simulink library "wt_blockset_v3"  (Simulink 6.0)
settings: Solver=ode45  SolverMode=SingleTasking  StartTime=0.0  StopTime=10.0  RelTol=1e-3
undefined symbols (not defined in the file): f1, get, j, Kmode, Type, u0
libraries: simulink_extras x12, simulink3 x5, simulink x4, dspinverses x1, dspmtrx3 x1, dspsnks4 x1
(part 4 of 7)

== system wt_blockset_v3/Control/WT Controller 2 MW DFIG/Pitch System ==
  In : Inport  Port=1  LatchInput=off
  Rate Limiter : RateLimiter  RisingSlewLimit=8  FallingSlewLimit=-8
  Saturation1 : Saturate  UpperLimit=90  LowerLimit=-90
  Out : Outport
  wires:
  Rate Limiter/1 -> Saturation1/1
  In/1 -> Rate Limiter/1
  Saturation1/1 -> Out/1

== system wt_blockset_v3/Control/WT Controller 2 MW DFIG/Power Controller ==
  Ref : Inport  Port=1  LatchInput=off
  Meas : Inport  Port=2  LatchInput=off
  Gain : Inport  Port=3  LatchInput=off
  1/T : Gain  Gain=1/Ti  SaturateOnIntegerOverflow=on
  Integrator : Integrator  InitialCondition=init_cond
  Limit Pitch : Saturate  UpperLimit=24  LowerLimit=0
  P1 : Gain  Gain=K  SaturateOnIntegerOverflow=on
  P2 : Gain  Orientation=left  Gain=ka  SaturateOnIntegerOverflow=on
  Product : Product  InputSameDT=on
  Sum1 : Sum  Inputs=|+-  SaturateOnIntegerOverflow=on  InputSameDT=on
  Sum2 : Sum  Inputs=++|  SaturateOnIntegerOverflow=on  InputSameDT=on
  Sum3 : Sum  Inputs=|+-  SaturateOnIntegerOverflow=on  InputSameDT=on
  Sum4 : Sum  Orientation=left  Inputs=+-|  SaturateOnIntegerOverflow=on  InputSameDT=on
  Out : Outport  InitialOutput=0
  wires:
  Limit Pitch/1 -> Sum4/2, Out/1
  Sum4/1 -> P2/1
  Sum2/1 -> Limit Pitch/1, Sum4/1
  P2/1 -> Sum1/2
  Meas/1 -> Sum3/2
  Ref/1 -> Sum3/1
  Sum3/1 -> P1/1
  1/T/1 -> Integrator/1
  Integrator/1 -> Sum2/2
  Sum1/1 -> 1/T/1
  P1/1 -> Product/1
  Product/1 -> Sum1/1, Sum2/1
  Gain/1 -> Product/2

== system wt_blockset_v3/Control/WT Controller 2 MW DFIG/Speed Controller ==
  ref : Inport  Port=1  LatchInput=off
  meas : Inport  Port=2  LatchInput=off
  1/T : Gain  Gain=1/Ti  SaturateOnIntegerOverflow=on
  Integrator : Integrator  InitialCondition=init_cond
  P1 : Gain  Gain=K  SaturateOnIntegerOverflow=on
  P2 : Gain  Orientation=left  Gain=ka  SaturateOnIntegerOverflow=on
  Saturation : Saturate  UpperLimit=maxim  LowerLimit=-maxim
  Sum1 : Sum  Inputs=|+-  SaturateOnIntegerOverflow=on  InputSameDT=on
  Sum2 : Sum  Inputs=++|  SaturateOnIntegerOverflow=on  InputSameDT=on
  Sum3 : Sum  Inputs=|+-  SaturateOnIntegerOverflow=on  InputSameDT=on
  Sum4 : Sum  Orientation=left  Inputs=+-|  SaturateOnIntegerOverflow=on  InputSameDT=on
  out : Outport  InitialOutput=0
  wires:
  Saturation/1 -> Sum4/2, out/1
  Sum4/1 -> P2/1
  Sum2/1 -> Saturation/1, Sum4/1
  P2/1 -> Sum1/2
  meas/1 -> Sum3/2
  P1/1 -> Sum2/1, Sum1/1
  ref/1 -> Sum3/1
  Sum3/1 -> P1/1
  1/T/1 -> Integrator/1
  Integrator/1 -> Sum2/2
  Sum1/1 -> 1/T/1

== system wt_blockset_v3/Electrical Machinery/C S-Function based  Models/ABC/abc Squirrel Cage Induction Machine ==
  us_UVW : Inport  Port=1  LatchInput=off
  omg_mec : Inport  Port=2  LatchInput=off
  Connection Type : Constant  Value=Type
  Demux : Demux  Outputs=[3 1]
  Mux : Mux  Inputs=[3 1]
  S-Function : S-Function  FunctionName=abc_scim_zcs  Parameters=stator rotor Lm p x0_init
  Switch : Switch  SaturateOnIntegerOverflow=on  InputSameDT=on
  mode : Gain  Gain=Kmode  SaturateOnIntegerOverflow=on
  phase ->line : Subsystem
  is_UVW : Outport
  Te : Outport  Port=2
  wires:
  Mux/1 -> S-Function/1
  S-Function/1 -> Demux/1
  us_UVW/1 -> mode/1
  omg_mec/1 -> Mux/2
  Demux/2 -> Te/1
  mode/1 -> Mux/1
  phase ->line/1(Out) -> Switch/3
  Connection Type/1 -> Switch/2
  Switch/1 -> is_UVW/1
  Demux/1 -> Switch/1, phase ->line/1(In)

== system wt_blockset_v3/Electrical Machinery/C S-Function based  Models/ABC/abc Wound Rotor Induction Machine ==
  us_UVW : Inport  Port=1  LatchInput=off
  ur_KLM : Inport  Port=2  LatchInput=off
  omg_mec : Inport  Port=3  LatchInput=off
  Connection Type : Constant  Value=Type
  Demux : Demux  Outputs=[3 3 1]
  Mux : Mux  Inputs=[3 3 1]
  S-Function : S-Function  FunctionName=abc_wrim_zcs  Parameters=stator rotor Lm p x0_init
  Switch : Switch  SaturateOnIntegerOverflow=on  InputSameDT=on
  mode : Gain  Gain=Kmode  SaturateOnIntegerOverflow=on
  phase ->line1 : Subsystem
  is_UVW : Outport
  ir_KLM : Outport  Port=2
  Te : Outport  Port=3
  wires:
  Mux/1 -> S-Function/1
  S-Function/1 -> Demux/1
  us_UVW/1 -> mode/1
  mode/1 -> Mux/1
  phase ->line1/1(Out) -> Switch/3
  Connection Type/1 -> Switch/2
  Switch/1 -> is_UVW/1
  Demux/1 -> Switch/1, phase ->line1/1(In)
  omg_mec/1 -> Mux/3
  ur_KLM/1 -> Mux/2
  Demux/3 -> Te/1
  Demux/2 -> ir_KLM/1

== system wt_blockset_v3/Electrical Machinery/C S-Function based  Models/DQ Salient-Pole Synchronous Machine ==
  us_UVW : Inport  Port=1  LatchInput=off
  uf : Inport  Port=2  LatchInput=off
  omg_mec : Inport  Port=3  LatchInput=off
  Demux : Demux  Outputs=[3 1 1]
  Mux : Mux  Inputs=[3 1 1]
  S-Function : S-Function  FunctionName=sp_sm_rot_mask  Parameters=stator_winding, field_winding, rotor_winding, mag_ind, p
  is_UVW : Outport  InitialOutput=0
  if : Outport  Port=2  InitialOutput=0
  Te : Outport  Port=3  InitialOutput=0
  wires:
  us_UVW/1 -> Mux/1
  uf/1 -> Mux/2
  omg_mec/1 -> Mux/3
  Demux/1 -> is_UVW/1
  Demux/2 -> if/1
  Demux/3 -> Te/1
  Mux/1 -> S-Function/1
  S-Function/1 -> Demux/1

== system wt_blockset_v3/Electrical Machinery/C S-Function based  Models/DQ Squirrel Cage Induction Machine ==
  us_UVW : Inport  Port=1  LatchInput=off
  omg_mec : Inport  Port=2  LatchInput=off
  Demux : Demux  Outputs=[3 1]
  Mux : Mux  Inputs=[3 1]
  S-Function : S-Function  FunctionName=dq_scim  Parameters=stator rotor Lm p x0_init
  is_UVW : Outport
  Te : Outport  Port=2
  wires:
  Demux/2 -> Te/1
  Demux/1 -> is_UVW/1
  omg_mec/1 -> Mux/2
  us_UVW/1 -> Mux/1
  S-Function/1 -> Demux/1
  Mux/1 -> S-Function/1

== system wt_blockset_v3/Electrical Machinery/C S-Function based  Models/DQ Wound Rotor Induction Machine ==
  us_UVW : Inport  Port=1  LatchInput=off
  ur_KLM : Inport  Port=2  LatchInput=off
  omg_mec : Inport  Port=3  LatchInput=off
  Demux : Demux  Outputs=[3 3 1]
  Mux : Mux  Inputs=[3 3 1]
  S-Function : S-Function  FunctionName=wr_imr  Parameters=stator rotor Lm p x0_init
  is_UVW : Outport
  ir_KLM : Outport  Port=2
  Te : Outport  Port=3
  wires:
  Demux/3 -> Te/1
  Demux/2 -> ir_KLM/1
  Demux/1 -> is_UVW/1
  omg_mec/1 -> Mux/3
  ur_KLM/1 -> Mux/2
  us_UVW/1 -> Mux/1
  S-Function/1 -> Demux/1
  Mux/1 -> S-Function/1

== system wt_blockset_v3/Electrical Machinery/Simulink Blocks  based Models/ABC/abc Squirell-Cage Induction Machine ==
  v_UVW : Inport  Port=1  LatchInput=off
  omg_mec : Inport  Port=2  LatchInput=off
  Connection Type : Constant  Value=Type
  Int_iA : Integrator  InitialCondition=init_cond(1)
  Int_iB : Integrator  InitialCondition=init_cond(2)
  Int_iC : Integrator  InitialCondition=init_cond(3)
  Int_ia : Integrator  InitialCondition=init_cond(4)
  Int_ib : Integrator  InitialCondition=init_cond(5)
  Int_ic : Integrator  InitialCondition=init_cond(6)
  Int_theta : Integrator  InitialCondition=init_cond(7)
  Mux : Mux  Inputs=[1 1 1 1 1 1 3 1 1]
  Selector i_UVW : Selector  Elements=[1 2 3]  InputPortWidth=11
  Switch : Switch  SaturateOnIntegerOverflow=on  InputSameDT=on
  Telm : Fcn  Expr=-p*Msr*((u(1)*u(4)+u(2)*u(5)+u(3)*u(6))*sin(u(11))+(u(1)*u(5)+u(2)*u(6)+u(3)*u(4))*sin(u(11)+dlt)+(u(1)*u(6)+u(2)*u(4)+u(3)*u(5))*sin(u(11)-dlt))
  diA : Fcn  Expr=-a11*u(1)-(a12+a13*u(10))*u(2)-(a12-a13*u(10))*u(3)-(a14*cos(u(11))-u(10)*sin(u(11))*a15)*u(4)-(a14*cos(u(11)+dlt)-u(10)*sin(u(11)+dlt)*a15)*u(5)-(a14*cos(u(11)-dlt)-u(10)*sin(u(11)-dlt)*a15)*u(6)+a16*u(7)+a17*(u(8)+u(9))
  diB : Fcn  Expr=-a11*u(2)-(a12-a13*u(10))*u(1)-(a12+a13*u(10))*u(3)-(a14*cos(u(11)-dlt)-u(10)*sin(u(11)-dlt)*a15)*u(4)-(a14*cos(u(11))-u(10)*sin(u(11))*a15)*u(5)-(a14*cos(u(11)+dlt)-u(10)*sin(u(11)+dlt)*a15)*u(6)+a16*u(8)+a17*(u(7)+u(9))
  diC : Fcn  Expr=-a11*u(3)-(a12+a13*u(10))*u(1)-(a12-a13*u(10))*u(2)-(a14*cos(u(11)+dlt)-u(10)*sin(u(11)+dlt)*a15)*u(4)-(a14*cos(u(11)-dlt)-u(10)*sin(u(11)-dlt)*a15)*u(5)-(a14*cos(u(11))-u(10)*sin(u(11))*a15)*u(6)+a16*u(9)+a17*(u(7)+u(8))
  dia : Fcn  Expr=-(a31*cos(u(11))-u(10)*sin(u(11))*a32)*u(1)-(a31*cos(u(11)-dlt)-u(10)*sin(u(11)-dlt)*a32)*u(2)-(a31*cos(u(11)+dlt)-u(10)*sin(u(11)+dlt)*a32)*u(3)-a33*u(4)-(a34-u(10)*a35)*u(5)-(a34+u(10)*a35)*u(6)+a36*(cos(u(11))*u(7)+cos(u(11)-dlt)*u(8)+cos(u(11)+dlt)*u(9))
  dib : Fcn  Expr=-(a31*cos(u(11)+dlt)-u(10)*sin(u(11)+dlt)*a32)*u(1)-(a31*cos(u(11))-u(10)*sin(u(11))*a32)*u(2)-(a31*cos(u(11)-dlt)-u(10)*sin(u(11)-dlt)*a32)*u(3)-a33*u(5)-(a34+u(10)*a35)*u(4)-(a34-u(10)*a35)*u(6)+a36*(cos(u(11)+dlt)*u(7)+cos(u(11))*u(8)+cos(u(11)-dlt)*u(9))
  dic : Fcn  Expr=-(a31*cos(u(11)-dlt)-u(10)*sin(u(11)-dlt)*a32)*u(1)-(a31*cos(u(11)+dlt)-u(10)*sin(u(11)+dlt)*a32)*u(2)-(a31*cos(u(11))-u(10)*sin(u(11))*a32)*u(3)-a33*u(6)-(a34-u(10)*a35)*u(4)-(a34+u(10)*a35)*u(5)+a36*(cos(u(11)-dlt)*u(7)+cos(u(11)+dlt)*u(8)+cos(u(11))*u(9))
  mode : Gain  Gain=Kmode  SaturateOnIntegerOverflow=on
  p : Gain  Gain=p  SaturateOnIntegerOverflow=on
  phase ->line : Subsystem
  i_UVW : Outport
  Te : Outport  Port=2
  wires:
  Mux/1 -> diA/1, diB/1, diC/1, dia/1, dib/1, dic/1, Selector i_UVW/1, Telm/1
  Int_iA/1 -> Mux/1  "iA"
  Int_iB/1 -> Mux/2  "iB"
  Int_iC/1 -> Mux/3  "iC"
  Int_ia/1 -> Mux/4  "ia"
  Int_ib/1 -> Mux/5  "ib"
  Int_ic/1 -> Mux/6  "ic"
  diA/1 -> Int_iA/1
  diB/1 -> Int_iB/1
  diC/1 -> Int_iC/1
  dia/1 -> Int_ia/1
  dib/1 -> Int_ib/1
  dic/1 -> Int_ic/1
  omg_mec/1 -> p/1
  p/1 -> Mux/8, Int_theta/1
  Int_theta/1 -> Mux/9
  Telm/1 -> Te/1
  v_UVW/1 -> mode/1
  Selector i_UVW/1 -> phase ->line/1(In), Switch/1
  mode/1 -> Mux/7
  phase ->line/1(Out) -> Switch/3
  Connection Type/1 -> Switch/2
  Switch/1 -> i_UVW/1

== system wt_blockset_v3/Electrical Machinery/Simulink Blocks  based Models/ABC/abc Wound Rotor Induction Machine ==
  v_UVW : Inport  Port=1  LatchInput=off
  v_KLM : Inport  Port=2  LatchInput=off
  omg_mec : Inport  Port=3  LatchInput=off
  Int_iA : Integrator  InitialCondition=init_cond(1)
  Int_iB : Integrator  InitialCondition=init_cond(2)
  Int_iC : Integrator  InitialCondition=init_cond(3)
  Int_ia : Integrator  InitialCondition=init_cond(4)
  Int_ib : Integrator  InitialCondition=init_cond(5)
  Int_ic : Integrator  InitialCondition=init_cond(6)
  Int_theta : Integrator  InitialCondition=init_cond(7)
  Mux : Mux  Inputs=[1 1 1 1 1 1 3 3 1 1]
  Selector i_KLM : Selector  Elements=[4 5 6]  InputPortWidth=14
  Selector i_UVW : Selector  Elements=[1 2 3]  InputPortWidth=14
  Telm : Fcn  Expr=-p*Msr*((u(1)*u(4)+u(2)*u(5)+u(3)*u(6))*sin(u(14))+(u(1)*u(5)+u(2)*u(6)+u(3)*u(4))*sin(u(14)+dlt)+(u(1)*u(6)+u(2)*u(4)+u(3)*u(5))*sin(u(14)-dlt))
  diA : Fcn  Expr=-a11*u(1)-(a12+a13*u(13))*u(2)-(a12-a13*u(13))*u(3)-(a14*cos(u(14))-u(13)*sin(u(14))*a15)*u(4)-(a14*cos(u(14)+dlt)-u(13)*sin(u(14)+dlt)*a15)*u(5)-(a14*cos(u(14)-dlt)-u(13)*sin(u(14)-dlt)*a15)*u(6)+a16*u(7)+a17*(u(8)+u(9))+a18*(cos(u(14))*u(10)+cos(u(14)+dlt)*u(11)+cos(u(14)-dlt)*u(12))
  diB : Fcn  Expr=-a11*u(2)-(a12-a13*u(13))*u(1)-(a12+a13*u(13))*u(3)-(a14*cos(u(14)-dlt)-u(13)*sin(u(14)-dlt)*a15)*u(4)-(a14*cos(u(14))-u(13)*sin(u(14))*a15)*u(5)-(a14*cos(u(14)+dlt)-u(13)*sin(u(14)+dlt)*a15)*u(6)+a16*u(8)+a17*(u(7)+u(9))+a18*(cos(u(14)-dlt)*u(10)+cos(u(14))*u(11)+cos(u(14)+dlt)*u(12))
  diC : Fcn  Expr=-a11*u(3)-(a12+a13*u(13))*u(1)-(a12-a13*u(13))*u(2)-(a14*cos(u(14)+dlt)-u(13)*sin(u(14)+dlt)*a15)*u(4)-(a14*cos(u(14)-dlt)-u(13)*sin(u(14)-dlt)*a15)*u(5)-(a14*cos(u(14))-u(13)*sin(u(14))*a15)*u(6)+a16*u(9)+a17*(u(7)+u(8))+a18*(cos(u(14)+dlt)*u(10)+cos(u(14)-dlt)*u(11)+cos(u(14))*u(12))
  dia : Fcn  Expr=-(a31*cos(u(14))-u(13)*sin(u(14))*a32)*u(1)-(a31*cos(u(14)-dlt)-u(13)*sin(u(14)-dlt)*a32)*u(2)-(a31*cos(u(14)+dlt)-u(13)*sin(u(14)+dlt)*a32)*u(3)-a33*u(4)-(a34-u(13)*a35)*u(5)-(a34+u(13)*a35)*u(6)+a36*(cos(u(14))*u(7)+cos(u(14)-dlt)*u(8)+cos(u(14)+dlt)*u(9))+a37*u(10)+a38*(u(11)+u(12))
  dib : Fcn  Expr=-(a31*cos(u(14)+dlt)-u(13)*sin(u(14)+dlt)*a32)*u(1)-(a31*cos(u(14))-u(13)*sin(u(14))*a32)*u(2)-(a31*cos(u(14)-dlt)-u(13)*sin(u(14)-dlt)*a32)*u(3)-a33*u(5)-(a34+u(13)*a35)*u(4)-(a34-u(13)*a35)*u(6)+a36*(cos(u(14)+dlt)*u(7)+cos(u(14))*u(8)+cos(u(14)-dlt)*u(9))+a37*u(11)+a38*(u(10)+u(12))
  dic : Fcn  Expr=-(a31*cos(u(14)-dlt)-u(13)*sin(u(14)-dlt)*a32)*u(1)-(a31*cos(u(14)+dlt)-u(13)*sin(u(14)+dlt)*a32)*u(2)-(a31*cos(u(14))-u(13)*sin(u(14))*a32)*u(3)-a33*u(6)-(a34-u(13)*a35)*u(4)-(a34+u(13)*a35)*u(5)+a36*(cos(u(14)-dlt)*u(7)+cos(u(14)+dlt)*u(8)+cos(u(14))*u(9))+a38*(u(10)+u(11))+a37*u(12)
  p : Gain  Gain=p  SaturateOnIntegerOverflow=on
  i_UVW : Outport
  i_KLM : Outport  Port=2
  Te : Outport  Port=3
  wires:
  v_UVW/1 -> Mux/7
  Telm/1 -> Te/1
  p/1 -> Int_theta/1, Mux/9
  omg_mec/1 -> p/1
  dic/1 -> Int_ic/1
  dib/1 -> Int_ib/1
  dia/1 -> Int_ia/1
  diC/1 -> Int_iC/1
  diB/1 -> Int_iB/1
  diA/1 -> Int_iA/1
  Int_ic/1 -> Mux/6  "ic"
  Int_ib/1 -> Mux/5  "ib"
  Int_ia/1 -> Mux/4  "ia"
  Int_iC/1 -> Mux/3  "iC"
  Int_iB/1 -> Mux/2  "iB"
  Int_iA/1 -> Mux/1  "iA"
  Mux/1 -> Selector i_UVW/1, Telm/1, Selector i_KLM/1, dic/1, dib/1, dia/1, diC/1, diB/1, diA/1
  Int_theta/1 -> Mux/10
  v_KLM/1 -> Mux/8
  Selector i_UVW/1 -> i_UVW/1
  Selector i_KLM/1 -> i_KLM/1

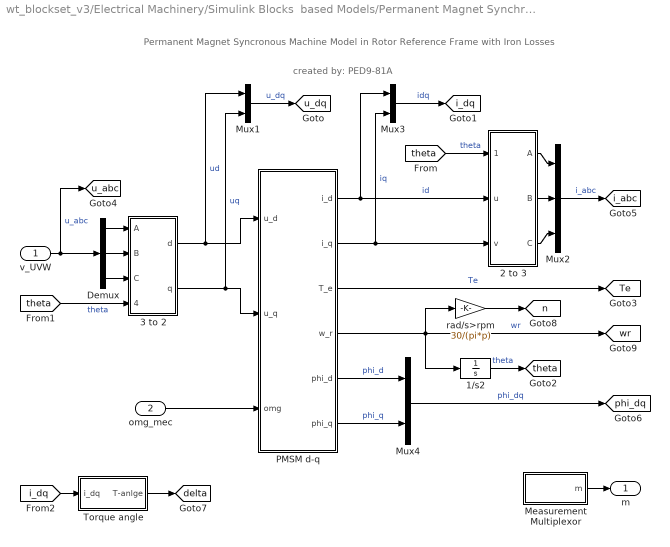
== system wt_blockset_v3/Electrical Machinery/Simulink Blocks  based Models/Permanent Magnet Synchronous Machine with iron losses ==
  note: Permanent Magnet Syncronous Machine Model
      | in Rotor Reference Frame with Iron Losses
  note: created by: PED9-81A
  v_UVW : Inport  Port=1  LatchInput=off
  omg_mec : Inport  Port=2  LatchInput=off
  1/s2 : Integrator
  "2 to 3 " : Subsystem
      mask Display: disp('2/3')
  3 to 2 : Subsystem
      mask Display: disp('3/2')
  Demux : Demux  Outputs=3
  Measurement Multiplexor : Subsystem
  Mux1 : Mux  Inputs=2
  Mux2 : Mux  Inputs=3
  Mux3 : Mux  Inputs=2
  Mux4 : Mux  Inputs=2
  PMSM d-q : Subsystem
  Torque angle : Subsystem
  rad/s>rpm : Gain  Gain=30/(pi*p)  SaturateOnIntegerOverflow=on
  m : Outport
  tag scope: Te=global, delta=global, i_abc=global, i_dq=global, n=global, phi_dq=global, theta=global, u_abc=global, u_dq=global, wr=global
  wires:
  3 to 2/2(q) -> PMSM d-q/2(u_q), Mux1/2  "uq"
  Demux/3 -> 3 to 2/3(C)
  Demux/2 -> 3 to 2/2(B)
  Demux/1 -> 3 to 2/1(A)
  3 to 2/1(d) -> PMSM d-q/1(u_d), Mux1/1  "ud"
  PMSM d-q/1(i_d) -> "2 to 3 "/2(u), Mux3/1  "id"
  PMSM d-q/2(i_q) -> "2 to 3 "/3(v), Mux3/2  "iq"
  "2 to 3 "/1(A) -> Mux2/1
  "2 to 3 "/2(B) -> Mux2/2
  "2 to 3 "/3(C) -> Mux2/3
  Mux1/1 -> [u_dq]  "u_dq"
  Mux3/1 -> [i_dq]  "idq"
  [theta] -> "2 to 3 "/1(theta)  "theta"
  [theta] -> 3 to 2/4(theta)  "theta"
  Mux2/1 -> [i_abc]  "i_abc"
  PMSM d-q/4(w_r) -> 1/s2/1, [wr], rad/s>rpm/1  "wr"
  1/s2/1 -> [theta]  "theta"
  v_UVW/1 -> Demux/1, [u_abc]  "u_abc"
  omg_mec/1 -> PMSM d-q/3(omg)
  PMSM d-q/5(phi_d) -> Mux4/1  "phi_d"
  PMSM d-q/6(phi_q) -> Mux4/2  "phi_q"
  Mux4/1 -> [phi_dq]  "phi_dq"
  [i_dq] -> Torque angle/1(i_dq)
  Torque angle/1(T-anlge) -> [delta]
  PMSM d-q/3(T_e) -> [Te]  "Te"
  rad/s>rpm/1 -> [n]
  Measurement Multiplexor/1(m) -> m/1

== system wt_blockset_v3/Electrical Machinery/Simulink Blocks  based Models/RMS Wound Rotor Induction Machine ==
  note: Comple steady state model for induction machine.
      | Deep-bar effect is taken into account
  Vs_c : Inport  Port=1  LatchInput=off
  Vr_c : Inport  Port=2  LatchInput=off
  omg_mec : Inport  Port=3  LatchInput=off
  " LU Inverse" : dspinverses/ LU Inverse
  Complex to Real-Imag : ComplexToRealImag  Output=Real
  Gain : Gain  Gain=3*p*Xm/omg_synch/2  SaturateOnIntegerOverflow=on
  Gain3 : Gain  Gain=p  SaturateOnIntegerOverflow=on
  Impedance Matrix : Subsystem
  Math Function : Math  Operator=conj  SaturateOnIntegerOverflow=on
  Matrix Concatenation : S-Function  FunctionName=smatrxcat  Parameters=numInports,catMethod  mask(Matrix Concatenation){numInports=2, catMethod=Vertical}
      mask prompts: numInports "Number of inputs:"; catMethod "Concatenation method:"
      mask help: Perform horizontal or vertical concatenation. 1-D vector input signals are treated as column vectors, i.e., [Mx1] matrices. The output is always a matrix.
      mask init:
      | xy = matrxcatmask('icon');
      mask StyleString: edit,popup(Horizontal|Vertical)
      mask Display:
      | plot(xy.x,xy.y);
      | text(0.15,0.86,xy.label);
  Matrix Multiply : dspmtrx3/Matrix Multiply  numInputPorts=2  OptimizationLevel=None
  Product : Product  Inputs=3  SaturateOnIntegerOverflow=on  InputSameDT=on
  Selector Ir : Selector  Elements=[2]  InputPortWidth=2
  Selector Is : Selector  Elements=[1]  InputPortWidth=2
  op : Constant  Value=j
  Is_c : Outport
  Ir_c : Outport  Port=2
  Te : Outport  Port=3
  wires:
  Gain3/1 -> Impedance Matrix/1(omg)
  Gain/1 -> Te/1
  Complex to Real-Imag/1 -> Gain/1
  op/1 -> Product/3
  Product/1 -> Complex to Real-Imag/1
  Selector Ir/1 -> Ir_c/1, Product/2
  Math Function/1 -> Product/1
  Selector Is/1 -> Is_c/1, Math Function/1
  Matrix Multiply/1 -> Selector Ir/1, Selector Is/1
  Matrix Concatenation/1 -> Matrix Multiply/2
  " LU Inverse"/1 -> Matrix Multiply/1
  Impedance Matrix/1(Z) -> " LU Inverse"/1
  omg_mec/1 -> Gain3/1  "slip"
  Vr_c/1 -> Matrix Concatenation/2
  Vs_c/1 -> Matrix Concatenation/1

== system wt_blockset_v3/Electrical Machinery/Simulink Blocks  based Models/RMS  Squirrel Cage Induction Machine ==
  Vs : Inport  Port=1  LatchInput=off
  omg_mec : Inport  Port=2  LatchInput=off
  Gain3 : Gain  Gain=p  SaturateOnIntegerOverflow=on
  Steady State Model : Subsystem
  Is : Outport  InitialOutput=0
  Te : Outport  Port=2  InitialOutput=0
  wires:
  Steady State Model/2(Iph) -> Is/1
  Steady State Model/1(Te) -> Te/1
  Gain3/1 -> Steady State Model/2(omg)
  Vs/1 -> Steady State Model/1(Vs)
  omg_mec/1 -> Gain3/1

== system wt_blockset_v3/Electrical Machinery/Simulink Blocks  based Models/Reduced Order Model Induction Machine ==
  vdq_s : Inport  Port=1  LatchInput=off
  vdq_r : Inport  Port=2  LatchInput=off
  omg_mec : Inport  Port=3  LatchInput=off
  Gain : Gain  Gain=Q  Multiplication=Matrix(K*u)  SaturateOnIntegerOverflow=on
  Mux : Mux  Inputs=[1 1 2 2 1]
  Mux1 : Mux  Inputs=[1 1 2]
  OpType : Gain  Gain=-1  SaturateOnIntegerOverflow=on
  Reshape : S-Function  FunctionName=sreshape  Parameters=OutputDimensionality, OutputDimensions  mask(Reshape){OutputDimensionality=Column vector, OutputDimensions=[1,1]}
      mask prompts: OutputDimensionality "Output dimensionality:"; OutputDimensions "Output dimensions:"
      mask help:
      | Change the dimensions of a vector or matrix input signal. Output
      |  - a one-dimensional array (vector),
      |  - a column vector (Mx1 matrix),
      |  - a row vector (1xN matrix), or
      |  - a matrix or vector with specified dimensions, e.g., [M, N] or [W].
      mask init:
      | s = reshapemask(gcb,'init');
      mask StyleString: popup(1-D array|Column vector|Row vector|Customize),edit
      mask CallbackString: reshapemask(gcb,'cbDimensionality')|
      mask Display: plot(s.x1,s.y1,s.xc,s.yc);
  Selector : Selector  Elements=[1 2]  InputPortWidth=7
  Te_dyn : Fcn  Expr=1.5*p*Lm*(u(2)*u(3)-u(1)*u(4))/D
  dfi_dr : Integrator  InitialCondition=init_cond(1)
  dfi_qr : Integrator  InitialCondition=init_cond(2)
  fi_dr : Fcn  Expr=tau_rm*(alpha*sigma_r-1/sigma_s)*u(1)+(alpha*omg_e*tau_rm*Lm/tau_sr+omg_e-u(7))*u(2)+alpha*omg_e*tau_rm*u(4)/(tau_sr^2)+alpha*tau_rm*u(3)/tau_sr+u(5)
  fi_ds : Fcn  Expr=alpha*(sigma_r*u(1)+omg_e*Lm/tau_sr*u(2)+omg_e*u(4)/(tau_sr^2)+u(3)/tau_sr)
  fi_qr : Fcn  Expr=-(alpha*omg_e*tau_rm*Lm/tau_sr+omg_e-u(7))*u(1)+tau_rm*(alpha*sigma_r-1/sigma_s)*u(2)+alpha*tau_rm*u(4)/tau_sr-alpha*omg_e*tau_rm*u(3)/(tau_sr^2)+u(6)
  fi_qs : Fcn  Expr=alpha*(-omg_e*Lm*u(1)/tau_sr+sigma_r*u(2)+u(4)/tau_sr-omg_e*u(3)/(tau_sr^2))
  p : Gain  Gain=p  SaturateOnIntegerOverflow=on
  sel_1 : Selector  Elements=[1 2]  InputPortWidth=4
  sel_2 : Selector  Elements=[3 4]  InputPortWidth=4
  idq_s : Outport
  idq_r : Outport  Port=2
  Te : Outport  Port=3
  wires:
  dfi_dr/1 -> Mux/1
  dfi_qr/1 -> Mux/2
  Mux/1 -> fi_dr/1, fi_qr/1, fi_ds/1, fi_qs/1, Selector/1
  fi_dr/1 -> dfi_dr/1
  fi_qr/1 -> dfi_qr/1
  fi_ds/1 -> Mux1/1
  fi_qs/1 -> Mux1/2
  Selector/1 -> Mux1/3
  Mux1/1 -> Te_dyn/1, Reshape/1
  Reshape/1 -> Gain/1
  p/1 -> Mux/5
  omg_mec/1 -> p/1
  vdq_s/1 -> OpType/1
  vdq_r/1 -> Mux/4
  Te_dyn/1 -> Te/1
  sel_1/1 -> idq_s/1
  Gain/1 -> sel_1/1, sel_2/1
  sel_2/1 -> idq_r/1
  OpType/1 -> Mux/3

== system wt_blockset_v3/Electrical Machinery/Simulink Blocks  based Models/Salient-Pole Synchronous Machine constant parameters ==
  note: Generalized model of synchronous machine in rotor reference frame
  vs_UVW : Inport  Port=1  LatchInput=off
  vf : Inport  Port=2  LatchInput=off
  omg_mec : Inport  Port=3  LatchInput=off
  Gain2 : Gain  Gain=p  SaturateOnIntegerOverflow=on
  Integrator1 : Integrator
  Mathematical model : Subsystem
  abc-dq : Subsystem
  Te : Outport  InitialOutput=0
  is_UVW : Outport  Port=2  InitialOutput=0
  tag scope: theta=global
  wires:
  vs_UVW/1 -> abc-dq/1(ABC)
  Integrator1/1 -> [theta]
  [theta] -> abc-dq/2(theta)
  abc-dq/1(DQ) -> Mathematical model/1(usdq)
  vf/1 -> Mathematical model/2(uf)
  Mathematical model/1(Te) -> Te/1
  omg_mec/1 -> Gain2/1
  Gain2/1 -> Mathematical model/3(omgr), Integrator1/1
  Mathematical model/2(is_UVW) -> is_UVW/1

== system wt_blockset_v3/Electrical Machinery/Simulink Blocks  based Models/Squirrel Cage Induction Machine constant parameters ==
  vs_UVW : Inport  Port=1  LatchInput=off
  omg_mec : Inport  Port=2  LatchInput=off
  Connection Type : Constant  Value=Type
  Derivatives : Subsystem
  Gain3 : Gain  Gain=p  SaturateOnIntegerOverflow=on
  Switch : Switch  SaturateOnIntegerOverflow=on  InputSameDT=on
  abc-dq : Subsystem
  dq / abc : Subsystem
  mode : Gain  Gain=Kmode  SaturateOnIntegerOverflow=on
  phase ->line : Subsystem
  is_UVW : Outport  InitialOutput=0
  Te : Outport  Port=2  InitialOutput=0
  wires:
  [theta] -> dq / abc/2(theta)
  Derivatives/1(idqs) -> dq / abc/1(DQ)
  Derivatives/2(Te) -> Te/1
  Gain3/1 -> Derivatives/2(omega)
  abc-dq/1(DQ) -> Derivatives/1(vdqs)
  vs_UVW/1 -> mode/1
  omg_mec/1 -> Gain3/1
  [theta] -> abc-dq/2(theta)
  mode/1 -> abc-dq/1(ABC)
  phase ->line/1(Out) -> Switch/3
  Connection Type/1 -> Switch/2
  Switch/1 -> is_UVW/1
  dq / abc/1(ABC) -> Switch/1, phase ->line/1(In)

== system wt_blockset_v3/Electrical Machinery/Simulink Blocks  based Models/Squirrel Cage  Induction Machine  with Deep Bar Effect ==
  vs_UVW : Inport  Port=1  LatchInput=off
  omg_mec : Inport  Port=2  LatchInput=off
  Connection Type : Constant  Value=Type
  Derivatives : Subsystem
  Gain3 : Gain  Gain=p  SaturateOnIntegerOverflow=on
  Subsystem1 : Subsystem
  Switch : Switch  SaturateOnIntegerOverflow=on  InputSameDT=on
  abc-dq : Subsystem
  mode : Gain  Gain=Kmode  SaturateOnIntegerOverflow=on
  phase ->line : Subsystem
  is_UVW : Outport  InitialOutput=0
  Te : Outport  Port=2  InitialOutput=0
  wires:
  [theta] -> Subsystem1/2(theta)
  Derivatives/1(idqs) -> Subsystem1/1(DQ)
  Derivatives/2(Te) -> Te/1
  Gain3/1 -> Derivatives/2(omega)
  abc-dq/1(DQ) -> Derivatives/1(vdqs)
  vs_UVW/1 -> mode/1
  omg_mec/1 -> Gain3/1
  [theta] -> abc-dq/2(theta)
  mode/1 -> abc-dq/1(ABC)
  phase ->line/1(Out) -> Switch/3
  Connection Type/1 -> Switch/2
  Switch/1 -> is_UVW/1
  Subsystem1/1(ABC) -> phase ->line/1(In), Switch/1

== system wt_blockset_v3/Electrical Machinery/Simulink Blocks  based Models/Wound Rotor Induction Machine constant parameters ==
  vs_UVW : Inport  Port=1  LatchInput=off
  vr_KLM : Inport  Port=2  LatchInput=off
  omg_mec : Inport  Port=3  LatchInput=off
  Constant : Constant  Value=0
  Constant1 : Constant  Value=0
  Gain1 : Gain  Gain=p  SaturateOnIntegerOverflow=on
  Subsystem1 : Subsystem
  Subsystem2 : Subsystem
  Voltage equations : Subsystem
  abc-dq : Subsystem
  abc-dq1 : Subsystem
  is_UVW : Outport  InitialOutput=0
  ir_KLM : Outport  Port=2  InitialOutput=0
  Te : Outport  Port=3  InitialOutput=0
  wires:
  Voltage equations/3(Te) -> Te/1
  Voltage equations/2(idqr) -> Subsystem2/1(DQ)
  abc-dq1/1(DQ) -> Voltage equations/2(vdqr)
  Subsystem2/1(ABC) -> ir_KLM/1
  Constant1/1 -> Subsystem2/2(theta)
  Subsystem1/1(ABC) -> is_UVW/1
  Constant/1 -> abc-dq1/2(theta)
  vr_KLM/1 -> abc-dq1/1(ABC)
  Gain1/1 -> Voltage equations/3(omega)
  omg_mec/1 -> Gain1/1
  [theta] -> Subsystem1/2(theta)
  Voltage equations/1(idqs) -> Subsystem1/1(DQ)
  abc-dq/1(DQ) -> Voltage equations/1(vdqs)
  vs_UVW/1 -> abc-dq/1(ABC)
  [theta] -> abc-dq/2(theta)

== system wt_blockset_v3/Electrical Machinery/Simulink Blocks  based Models/Wound Rotor Induction Machine with Deep Bar Effect  ==
  vs_UVW : Inport  Port=1  LatchInput=off
  vr_KLM : Inport  Port=2  LatchInput=off
  omg_mec : Inport  Port=3  LatchInput=off
  Constant : Constant  Value=0
  Constant1 : Constant  Value=0
  Gain1 : Gain  Gain=p  SaturateOnIntegerOverflow=on
  Subsystem1 : Subsystem
  Subsystem2 : Subsystem
  Voltage equations : Subsystem
  abc-dq : Subsystem
  abc-dq1 : Subsystem
  is_UVW : Outport  InitialOutput=0
  ir_KLM : Outport  Port=2  InitialOutput=0
  Te : Outport  Port=3  InitialOutput=0
  wires:
  Voltage equations/3(Te) -> Te/1
  Voltage equations/2(idqr) -> Subsystem2/1(DQ)
  abc-dq1/1(DQ) -> Voltage equations/2(vdqr)
  Subsystem2/1(ABC) -> ir_KLM/1
  Constant1/1 -> Subsystem2/2(theta)
  Subsystem1/1(ABC) -> is_UVW/1
  Constant/1 -> abc-dq1/2(theta)
  vr_KLM/1 -> abc-dq1/1(ABC)
  Gain1/1 -> Voltage equations/3(omega)
  omg_mec/1 -> Gain1/1
  [theta] -> Subsystem1/2(theta)
  Voltage equations/1(idqs) -> Subsystem1/1(DQ)
  abc-dq/1(DQ) -> Voltage equations/1(vdqs)
  vs_UVW/1 -> abc-dq/1(ABC)
  [theta] -> abc-dq/2(theta)

== system wt_blockset_v3/Grid Models/3-ph line 2/break algebraic loop1 ==
  In1 : Inport  Port=1  LatchInput=off
  Init_cond : Constant  Value=x0
  Integrator : Integrator  InitialConditionSource=external
  K : Gain  Gain=K
  Sum : Sum  Inputs=|+-
  T : Gain  Gain=1/T
  Out1 : Outport
  wires:
  Sum/1 -> T/1
  T/1 -> Integrator/1
  Integrator/1 -> Sum/2, Out1/1
  Init_cond/1 -> Integrator/2
  K/1 -> Sum/1
  In1/1 -> K/1

== system wt_blockset_v3/Grid Models/3-phase 3 limb  C S-Function/phase->line2 ==
  in : Inport  Port=1  LatchInput=off
  Mux1 : Mux  Inputs=3
  ab : Fcn  Expr=u(1)-u(3)
  bc : Fcn  Expr=u(2)-u(1)
  ca : Fcn  Expr=u(3)-u(2)
  out : Outport
  wires:
  in/1 -> bc/1, ca/1, ab/1
  Mux1/1 -> out/1
  ca/1 -> Mux1/3
  bc/1 -> Mux1/2
  ab/1 -> Mux1/1

== system wt_blockset_v3/Grid Models/3-phase 3 limb  Transformer/phase->line2 ==
  in : Inport  Port=1  LatchInput=off
  Mux1 : Mux  Inputs=3
  ab : Fcn  Expr=u(1)-u(3)
  bc : Fcn  Expr=u(2)-u(1)
  ca : Fcn  Expr=u(3)-u(2)
  out : Outport
  wires:
  ab/1 -> Mux1/1
  bc/1 -> Mux1/2
  ca/1 -> Mux1/3
  Mux1/1 -> out/1
  in/1 -> ab/1, ca/1, bc/1

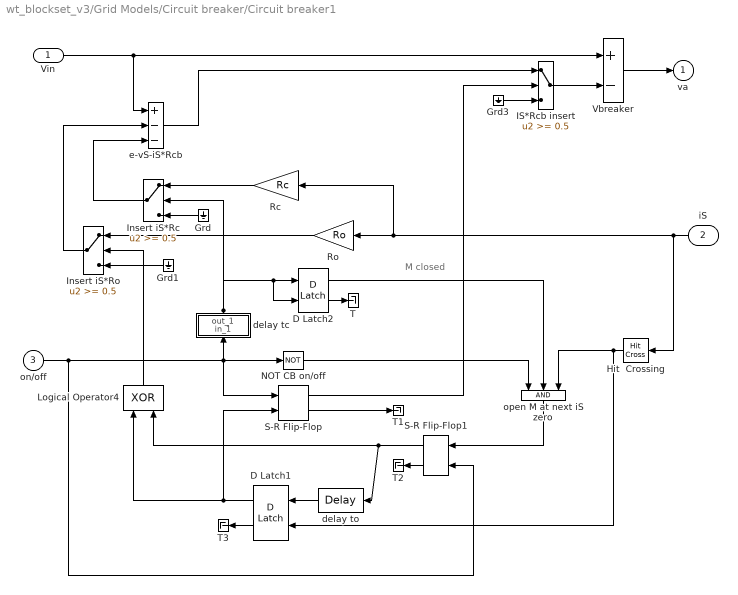
== system wt_blockset_v3/Grid Models/Circuit breaker/Circuit breaker1 ==
  note: M closed
  Vin : Inport  Port=1  LatchInput=off
  iS : Inport  Orientation=left  Port=2  LatchInput=off
  on/off : Inport  Port=3  LatchInput=off
  D Latch1 : simulink_extras/Flip Flops/D Latch  Orientation=left
  D Latch2 : simulink_extras/Flip Flops/D Latch
  Grd : Ground  Orientation=left
  Grd1 : Ground  Orientation=left
  Grd3 : Ground
  Hit  Crossing : HitCross  Orientation=left
  IS*Rcb insert : Switch  Threshold=0.5  SaturateOnIntegerOverflow=on  InputSameDT=on
  Insert iS*Rc : Switch  Orientation=left  Threshold=0.5  SaturateOnIntegerOverflow=on  InputSameDT=on
  Insert iS*Ro : Switch  Orientation=left  Threshold=0.5  SaturateOnIntegerOverflow=on  InputSameDT=on
  Logical Operator4 : Logic  Orientation=up  Operator=XOR
  NOT CB on/off : Logic  Operator=NOT  Inputs=1
  Rc : Gain  Orientation=left  Gain=Rc  SaturateOnIntegerOverflow=on
  Ro : Gain  Orientation=left  Gain=Ro  SaturateOnIntegerOverflow=on
  S-R Flip-Flop : simulink_extras/Flip Flops/S-R Flip-Flop  initial_condition=0
  S-R Flip-Flop1 : simulink_extras/Flip Flops/S-R Flip-Flop  Orientation=left  initial_condition=0
  T{,1..3} (4 alike) : Terminator
  Vbreaker : Sum  Inputs=+-  SaturateOnIntegerOverflow=on  InputSameDT=on
  delay tc : Subsystem  Orientation=up
  delay to : TransportDelay  Orientation=left  DelayTime=to  BufferSize=20000
  e-vS-iS*Rcb : Sum  Inputs=+--  SaturateOnIntegerOverflow=on  InputSameDT=on
  open M at next iS zero : Logic  Orientation=down  Inputs=3
  va : Outport
  wires:
  Ro/1 -> Insert iS*Ro/1
  e-vS-iS*Rcb/1 -> IS*Rcb insert/1
  Rc/1 -> Insert iS*Rc/1
  Insert iS*Ro/1 -> e-vS-iS*Rcb/2
  Insert iS*Rc/1 -> e-vS-iS*Rcb/3
  on/off/1 -> NOT CB on/off/1, S-R Flip-Flop1/2, delay tc/1(in_1), S-R Flip-Flop/1
  delay tc/1(out_1) -> D Latch2/1, D Latch2/2, Insert iS*Rc/2
  Logical Operator4/1 -> Insert iS*Ro/2
  Grd/1 -> Insert iS*Rc/3
  Grd1/1 -> Insert iS*Ro/3
  D Latch2/2 -> T/1
  delay to/1 -> D Latch1/1
  S-R Flip-Flop1/1 -> Logical Operator4/2, delay to/1
  S-R Flip-Flop1/2 -> T2/1
  Hit  Crossing/1 -> open M at next iS zero/3, D Latch1/2
  D Latch1/2 -> T3/1
  D Latch1/1 -> Logical Operator4/1, S-R Flip-Flop/2
  D Latch2/1 -> open M at next iS zero/2
  NOT CB on/off/1 -> open M at next iS zero/1
  open M at next iS zero/1 -> S-R Flip-Flop1/1
  Vbreaker/1 -> va/1
  IS*Rcb insert/1 -> Vbreaker/2
  Grd3/1 -> IS*Rcb insert/3
  Vin/1 -> Vbreaker/1, e-vS-iS*Rcb/1
  iS/1 -> Ro/1, Rc/1, Hit  Crossing/1
  S-R Flip-Flop/2 -> T1/1
  S-R Flip-Flop/1 -> IS*Rcb insert/2

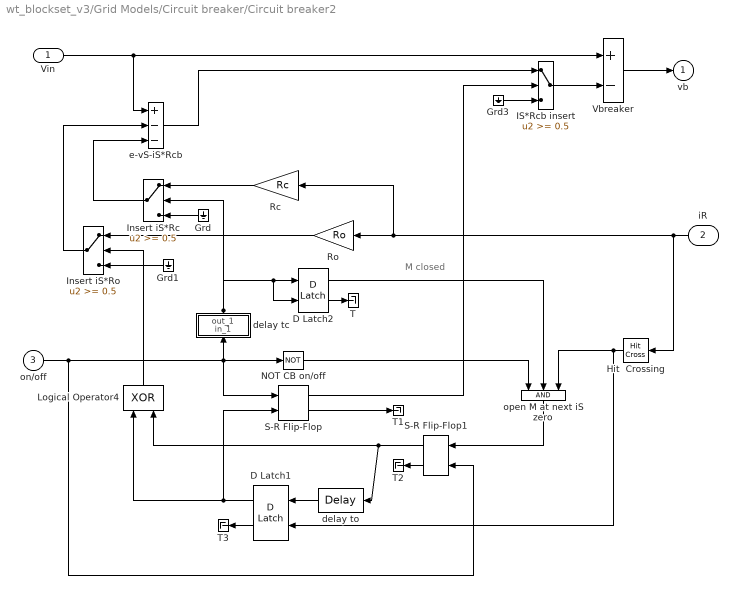
== system wt_blockset_v3/Grid Models/Circuit breaker/Circuit breaker2 ==
  note: M closed
  Vin : Inport  Port=1  LatchInput=off
  iR : Inport  Orientation=left  Port=2  LatchInput=off
  on/off : Inport  Port=3  LatchInput=off
  D Latch1 : simulink_extras/Flip Flops/D Latch  Orientation=left
  D Latch2 : simulink_extras/Flip Flops/D Latch
  Grd : Ground  Orientation=left
  Grd1 : Ground  Orientation=left
  Grd3 : Ground
  Hit  Crossing : HitCross  Orientation=left
  IS*Rcb insert : Switch  Threshold=0.5  SaturateOnIntegerOverflow=on  InputSameDT=on
  Insert iS*Rc : Switch  Orientation=left  Threshold=0.5  SaturateOnIntegerOverflow=on  InputSameDT=on
  Insert iS*Ro : Switch  Orientation=left  Threshold=0.5  SaturateOnIntegerOverflow=on  InputSameDT=on
  Logical Operator4 : Logic  Orientation=up  Operator=XOR
  NOT CB on/off : Logic  Operator=NOT  Inputs=1
  Rc : Gain  Orientation=left  Gain=Rc  SaturateOnIntegerOverflow=on
  Ro : Gain  Orientation=left  Gain=Ro  SaturateOnIntegerOverflow=on
  S-R Flip-Flop : simulink_extras/Flip Flops/S-R Flip-Flop  initial_condition=0
  S-R Flip-Flop1 : simulink_extras/Flip Flops/S-R Flip-Flop  Orientation=left  initial_condition=0
  T{,1..3} (4 alike) : Terminator
  Vbreaker : Sum  Inputs=+-  SaturateOnIntegerOverflow=on  InputSameDT=on
  delay tc : Subsystem  Orientation=up
  delay to : TransportDelay  Orientation=left  DelayTime=to  BufferSize=20000
  e-vS-iS*Rcb : Sum  Inputs=+--  SaturateOnIntegerOverflow=on  InputSameDT=on
  open M at next iS zero : Logic  Orientation=down  Inputs=3
  vb : Outport
  wires:
  S-R Flip-Flop/1 -> IS*Rcb insert/2
  S-R Flip-Flop/2 -> T1/1
  iR/1 -> Hit  Crossing/1, Rc/1, Ro/1
  Vin/1 -> e-vS-iS*Rcb/1, Vbreaker/1
  Grd3/1 -> IS*Rcb insert/3
  IS*Rcb insert/1 -> Vbreaker/2
  Vbreaker/1 -> vb/1
  open M at next iS zero/1 -> S-R Flip-Flop1/1
  NOT CB on/off/1 -> open M at next iS zero/1
  D Latch2/1 -> open M at next iS zero/2
  D Latch1/1 -> S-R Flip-Flop/2, Logical Operator4/1
  D Latch1/2 -> T3/1
  Hit  Crossing/1 -> D Latch1/2, open M at next iS zero/3
  S-R Flip-Flop1/2 -> T2/1
  S-R Flip-Flop1/1 -> delay to/1, Logical Operator4/2
  delay to/1 -> D Latch1/1
  D Latch2/2 -> T/1
  Grd1/1 -> Insert iS*Ro/3
  Grd/1 -> Insert iS*Rc/3
  Logical Operator4/1 -> Insert iS*Ro/2
  delay tc/1(out_1) -> Insert iS*Rc/2, D Latch2/2, D Latch2/1
  on/off/1 -> S-R Flip-Flop/1, delay tc/1(in_1), S-R Flip-Flop1/2, NOT CB on/off/1
  Insert iS*Rc/1 -> e-vS-iS*Rcb/3
  Insert iS*Ro/1 -> e-vS-iS*Rcb/2
  Rc/1 -> Insert iS*Rc/1
  e-vS-iS*Rcb/1 -> IS*Rcb insert/1
  Ro/1 -> Insert iS*Ro/1

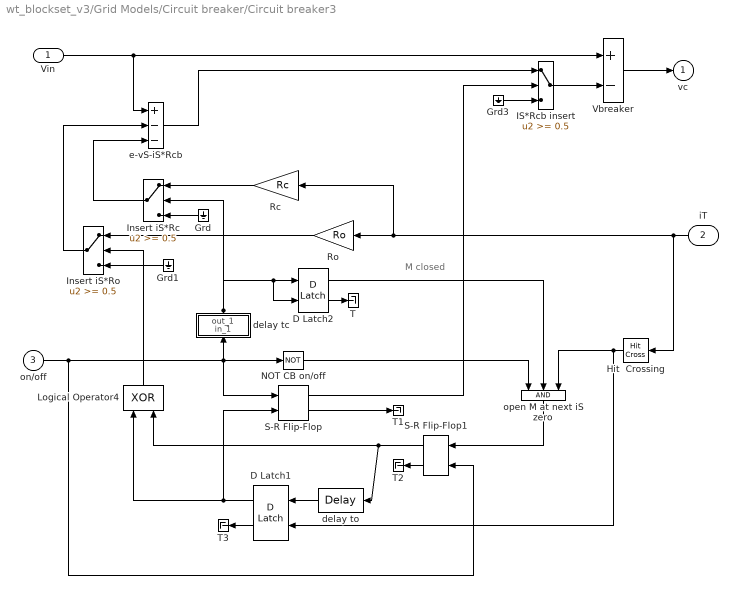
== system wt_blockset_v3/Grid Models/Circuit breaker/Circuit breaker3 ==
  note: M closed
  Vin : Inport  Port=1  LatchInput=off
  iT : Inport  Orientation=left  Port=2  LatchInput=off
  on/off : Inport  Port=3  LatchInput=off
  D Latch1 : simulink_extras/Flip Flops/D Latch  Orientation=left
  D Latch2 : simulink_extras/Flip Flops/D Latch
  Grd : Ground  Orientation=left
  Grd1 : Ground  Orientation=left
  Grd3 : Ground
  Hit  Crossing : HitCross  Orientation=left
  IS*Rcb insert : Switch  Threshold=0.5  SaturateOnIntegerOverflow=on  InputSameDT=on
  Insert iS*Rc : Switch  Orientation=left  Threshold=0.5  SaturateOnIntegerOverflow=on  InputSameDT=on
  Insert iS*Ro : Switch  Orientation=left  Threshold=0.5  SaturateOnIntegerOverflow=on  InputSameDT=on
  Logical Operator4 : Logic  Orientation=up  Operator=XOR
  NOT CB on/off : Logic  Operator=NOT  Inputs=1
  Rc : Gain  Orientation=left  Gain=Rc  SaturateOnIntegerOverflow=on
  Ro : Gain  Orientation=left  Gain=Ro  SaturateOnIntegerOverflow=on
  S-R Flip-Flop : simulink_extras/Flip Flops/S-R Flip-Flop  initial_condition=0
  S-R Flip-Flop1 : simulink_extras/Flip Flops/S-R Flip-Flop  Orientation=left  initial_condition=0
  T{,1..3} (4 alike) : Terminator
  Vbreaker : Sum  Inputs=+-  SaturateOnIntegerOverflow=on  InputSameDT=on
  delay tc : Subsystem  Orientation=up
  delay to : TransportDelay  Orientation=left  DelayTime=to  BufferSize=20000
  e-vS-iS*Rcb : Sum  Inputs=+--  SaturateOnIntegerOverflow=on  InputSameDT=on
  open M at next iS zero : Logic  Orientation=down  Inputs=3
  vc : Outport
  wires:
  Ro/1 -> Insert iS*Ro/1
  e-vS-iS*Rcb/1 -> IS*Rcb insert/1
  Rc/1 -> Insert iS*Rc/1
  Insert iS*Ro/1 -> e-vS-iS*Rcb/2
  Insert iS*Rc/1 -> e-vS-iS*Rcb/3
  on/off/1 -> NOT CB on/off/1, S-R Flip-Flop1/2, delay tc/1(in_1), S-R Flip-Flop/1
  delay tc/1(out_1) -> D Latch2/1, D Latch2/2, Insert iS*Rc/2
  Logical Operator4/1 -> Insert iS*Ro/2
  Grd/1 -> Insert iS*Rc/3
  Grd1/1 -> Insert iS*Ro/3
  D Latch2/2 -> T/1
  delay to/1 -> D Latch1/1
  S-R Flip-Flop1/1 -> Logical Operator4/2, delay to/1
  S-R Flip-Flop1/2 -> T2/1
  Hit  Crossing/1 -> open M at next iS zero/3, D Latch1/2
  D Latch1/2 -> T3/1
  D Latch1/1 -> Logical Operator4/1, S-R Flip-Flop/2
  D Latch2/1 -> open M at next iS zero/2
  NOT CB on/off/1 -> open M at next iS zero/1
  open M at next iS zero/1 -> S-R Flip-Flop1/1
  Vbreaker/1 -> vc/1
  IS*Rcb insert/1 -> Vbreaker/2
  Grd3/1 -> IS*Rcb insert/3
  Vin/1 -> Vbreaker/1, e-vS-iS*Rcb/1
  iT/1 -> Ro/1, Rc/1, Hit  Crossing/1
  S-R Flip-Flop/2 -> T1/1
  S-R Flip-Flop/1 -> IS*Rcb insert/2

== system wt_blockset_v3/Grid Models/GRID 2/Enabled and Triggered Subsystem ==
  In1 : Inport  Port=1  LatchInput=off
  Enable : EnablePort
  Trigger : TriggerPort  TriggerType=falling
  Out1 : Outport
  wires:
  In1/1 -> Out1/1

== system wt_blockset_v3/Grid Models/GRID 2/coeff ==
  In1 : Inport  Port=1  LatchInput=off
  Demux : Demux  Outputs=3
  Mux1 : Mux  Inputs=3
  Transfer Fcn : TransferFcn  Numerator=[1 0]  Denominator=[N 1]
  Transfer Fcn1 : TransferFcn  Numerator=[1 0]  Denominator=[N 1]
  Transfer Fcn2 : TransferFcn  Numerator=[1 0]  Denominator=[N 1]
  Out1 : Outport
  wires:
  Transfer Fcn/1 -> Mux1/1
  Transfer Fcn1/1 -> Mux1/2
  Transfer Fcn2/1 -> Mux1/3
  Demux/1 -> Transfer Fcn/1
  Demux/2 -> Transfer Fcn1/1
  Demux/3 -> Transfer Fcn2/1
  In1/1 -> Demux/1
  Mux1/1 -> Out1/1

== system wt_blockset_v3/Grid Models/GRID 2/short_path ==
  In1 : Inport  Orientation=left  Port=1  LatchInput=off
  Demux : Demux  Orientation=left  Outputs=3
  Gain1 : Gain  Orientation=left  Gain=1/Lf  SaturateOnIntegerOverflow=on
  Gain2 : Gain  Gain=Rf  SaturateOnIntegerOverflow=on
  Gain5 : Gain  Orientation=left  Gain=1/Lf  SaturateOnIntegerOverflow=on
  Gain6 : Gain  Gain=Rf  SaturateOnIntegerOverflow=on
  Integrator1 : Integrator  Orientation=left
  Integrator2 : Integrator  Orientation=left
  Mux : Mux  Orientation=left  Inputs=3
  Sum : Sum  Orientation=left  Inputs=--|
  Sum1 : Sum  Orientation=left  Inputs=|+-  SaturateOnIntegerOverflow=on  InputSameDT=on
  Sum3 : Sum  Orientation=left  Inputs=|+-  SaturateOnIntegerOverflow=on  InputSameDT=on
  Terminator : Terminator
  Out1 : Outport  Orientation=left
  wires:
  Sum3/1 -> Gain5/1
  Gain5/1 -> Integrator1/1
  Integrator1/1 -> Gain6/1, Mux/1, Sum/1
  Gain6/1 -> Sum3/2
  Demux/1 -> Sum3/1
  Sum1/1 -> Gain1/1
  Gain1/1 -> Integrator2/1
  Integrator2/1 -> Gain2/1, Mux/2, Sum/2
  Gain2/1 -> Sum1/2
  Demux/2 -> Sum1/1
  Mux/1 -> Out1/1
  Sum/1 -> Mux/3
  In1/1 -> Demux/1
  Demux/3 -> Terminator/1

== system wt_blockset_v3/Grid Models/Harmonic Voltage Source/Phase A ==
  Input : Inport  Port=1  LatchInput=off
  Constant1 : Constant  Value=[gama_0;0;0;0;0;0;0]
  Constant2 : Constant  Value=0
  Demux : Demux  Outputs=2
  Product : Product  SaturateOnIntegerOverflow=on
  Selector : Selector  Elements=[1]  InputPortWidth=7
  Sum1 : Sum  Inputs=|++  SaturateOnIntegerOverflow=on
  Sum3 : Sum  Inputs=|++  SaturateOnIntegerOverflow=on
  Sum4 : Sum  Inputs=1  SaturateOnIntegerOverflow=on
  Trigonometric Function : Trigonometry
  amplitudes : Gain  Gain=sqrt(2)*[1;0.05; 0.06; 0.05;0.015;0.035;0.03]  SaturateOnIntegerOverflow=on
  enable : Gain  Gain=[1; h3;h5;h7;h9;h11;h13]  SaturateOnIntegerOverflow=on
  order : Gain  Gain=[1;3;5;7;9;11;13]  SaturateOnIntegerOverflow=on
  v_harm : Outport
  tag scope: gama=global
  wires:
  Sum3/1 -> order/1
  Product/1 -> enable/1
  Sum4/1 -> v_harm/1
  Constant2/1 -> Sum3/2
  Trigonometric Function/1 -> Product/2
  amplitudes/1 -> Product/1
  order/1 -> Sum1/1
  Constant1/1 -> Sum1/2
  Input/1 -> Demux/1
  Demux/1 -> amplitudes/1
  Demux/2 -> Sum3/1
  enable/1 -> Sum4/1
  Selector/1 -> [gama]
  Sum1/1 -> Trigonometric Function/1, Selector/1

== system wt_blockset_v3/Grid Models/Harmonic Voltage Source/Phase B ==
  Input : Inport  Port=1  LatchInput=off
  Constant1 : Constant  Value=[gama_0;0;0;0;0;0;0]
  Constant2 : Constant  Value=-2*pi/3
  Demux : Demux  Outputs=2
  Product : Product  SaturateOnIntegerOverflow=on
  Sum1 : Sum  Inputs=|++  SaturateOnIntegerOverflow=on
  Sum3 : Sum  Inputs=|++  SaturateOnIntegerOverflow=on
  Sum4 : Sum  Inputs=1  SaturateOnIntegerOverflow=on
  Trigonometric Function : Trigonometry
  amplitudes : Gain  Gain=sqrt(2)*[1;0.05; 0.06; 0.05;0.015;0.035;0.03]  SaturateOnIntegerOverflow=on
  enable : Gain  Gain=[1; h3;h5;h7;h9;h11;h13]  SaturateOnIntegerOverflow=on
  order : Gain  Gain=[1;3;5;7;9;11;13]  SaturateOnIntegerOverflow=on
  v_harm : Outport
  wires:
  Demux/2 -> Sum3/1
  Demux/1 -> amplitudes/1
  Input/1 -> Demux/1
  Constant1/1 -> Sum1/2
  Sum1/1 -> Trigonometric Function/1
  order/1 -> Sum1/1
  amplitudes/1 -> Product/1
  Trigonometric Function/1 -> Product/2
  Constant2/1 -> Sum3/2
  Sum4/1 -> v_harm/1
  Product/1 -> enable/1
  Sum3/1 -> order/1
  enable/1 -> Sum4/1

== system wt_blockset_v3/Grid Models/Harmonic Voltage Source/Phase C ==
  Input : Inport  Port=1  LatchInput=off
  Constant1 : Constant  Value=[gama_0;0;0;0;0;0;0]
  Constant2 : Constant  Value=+2*pi/3
  Demux : Demux  Outputs=2
  Product : Product  SaturateOnIntegerOverflow=on
  Sum1 : Sum  Inputs=|++  SaturateOnIntegerOverflow=on
  Sum3 : Sum  Inputs=|++  SaturateOnIntegerOverflow=on
  Sum4 : Sum  Inputs=1  SaturateOnIntegerOverflow=on
  Trigonometric Function : Trigonometry
  amplitudes : Gain  Gain=sqrt(2)*[1;0.05; 0.06; 0.05;0.015;0.035;0.03]  SaturateOnIntegerOverflow=on
  enable : Gain  Gain=[1; h3;h5;h7;h9;h11;h13]  SaturateOnIntegerOverflow=on
  order : Gain  Gain=[1;3;5;7;9;11;13]  SaturateOnIntegerOverflow=on
  v_harm : Outport
  wires:
  Sum3/1 -> order/1
  Product/1 -> enable/1
  Sum4/1 -> v_harm/1
  Constant2/1 -> Sum3/2
  Trigonometric Function/1 -> Product/2
  amplitudes/1 -> Product/1
  order/1 -> Sum1/1
  Sum1/1 -> Trigonometric Function/1
  Constant1/1 -> Sum1/2
  Input/1 -> Demux/1
  Demux/1 -> amplitudes/1
  Demux/2 -> Sum3/1
  enable/1 -> Sum4/1

== system wt_blockset_v3/Measurements/Period/Sample and Hold ==
  In : Inport  Port=1  LatchInput=off
  Trigger : TriggerPort
  Zero-Order Hold : ZeroOrderHold  SampleTime=-1
  Out : Outport  InitialOutput=initCond
  wires:
  In/1 -> Zero-Order Hold/1
  Zero-Order Hold/1 -> Out/1

== system wt_blockset_v3/Measurements/Period/Sample and Hold1 ==
  In : Inport  Port=1  LatchInput=off
  Trigger : TriggerPort  TriggerType=falling
  Zero-Order Hold : ZeroOrderHold  SampleTime=-1
  Out : Outport  InitialOutput=initCond
  wires:
  In/1 -> Zero-Order Hold/1
  Zero-Order Hold/1 -> Out/1

== system wt_blockset_v3/Measurements/Phase Locked Loop/PI anti wind-up2 ==
  ref : Inport  Port=1  LatchInput=off
  1/T : Gain  Gain=1/Ti  SaturateOnIntegerOverflow=on
  Integrator : Integrator  InitialCondition=init_cond
  P1 : Gain  Gain=K  SaturateOnIntegerOverflow=on
  P2 : Gain  Orientation=left  Gain=ka  SaturateOnIntegerOverflow=on
  Saturation : Saturate  UpperLimit=maxim  LowerLimit=-maxim
  Sum1 : Sum  Inputs=|+-  SaturateOnIntegerOverflow=on  InputSameDT=on
  Sum2 : Sum  Inputs=++|  SaturateOnIntegerOverflow=on  InputSameDT=on
  Sum4 : Sum  Orientation=left  Inputs=+-|  SaturateOnIntegerOverflow=on  InputSameDT=on
  out : Outport  InitialOutput=0
  wires:
  Saturation/1 -> Sum4/2, out/1
  Sum4/1 -> P2/1
  Sum2/1 -> Saturation/1, Sum4/1
  P1/1 -> Sum2/1, Sum1/1
  ref/1 -> P1/1
  1/T/1 -> Integrator/1
  Integrator/1 -> Sum2/2
  Sum1/1 -> 1/T/1
  P2/1 -> Sum1/2

== system wt_blockset_v3/Mechanical Components/Wind Model SB-1/Kaimal_Filter_1 ==
  in_1 : Inport  Port=1  LatchInput=off
  Gain : Gain  Gain=trans/sqrt(2)  SaturateOnIntegerOverflow=on
  Transfer Fcn : TransferFcn  Numerator=[0.0182*c^2 1.3653*c 0.9846]  Denominator=[1.3463*c^2 3.7593*c 1]
  Unit Delay : UnitDelay  SampleTime=T_sample
  out_1 : Outport
  wires:
  Unit Delay/1 -> Transfer Fcn/1
  Gain/1 -> out_1/1
  in_1/1 -> Unit Delay/1
  Transfer Fcn/1 -> Gain/1

== system wt_blockset_v3/Mechanical Components/Wind Model SB-1/Kaimal_Filter_2 ==
  in_1 : Inport  Port=1  LatchInput=off
  Gain : Gain  Gain=trans/sqrt(2)  SaturateOnIntegerOverflow=on
  Transfer Function : TransferFcn  Numerator=[0.0182*c^2 1.3653*c 0.9846]  Denominator=[1.3463*c^2 3.7593*c 1]
  Unit Delay : UnitDelay  SampleTime=T_sample
  out_1 : Outport
  wires:
  Unit Delay/1 -> Transfer Function/1
  Gain/1 -> out_1/1
  in_1/1 -> Unit Delay/1
  Transfer Function/1 -> Gain/1

== system wt_blockset_v3/Mechanical Components/Wind Model SB-1/Kaimal_Filter_3 ==
  in_1 : Inport  Port=1  LatchInput=off
  Gain : Gain  Gain=trans/sqrt(2)  SaturateOnIntegerOverflow=on
  Transfer Fcn : TransferFcn  Numerator=[0.0182*c^2 1.3653*c 0.9846]  Denominator=[1.3463*c^2 3.7593*c 1]
  Unit Delay : UnitDelay  SampleTime=T_sample
  out_1 : Outport
  wires:
  Unit Delay/1 -> Transfer Fcn/1
  Gain/1 -> out_1/1
  in_1/1 -> Unit Delay/1
  Transfer Fcn/1 -> Gain/1

== system wt_blockset_v3/Mechanical Components/Wind Model SB-1/White Noise_1 ==
  Gain : Gain  Gain=[sqrt(Cov)]/[sqrt(Ts)]  SaturateOnIntegerOverflow=on
  White Noise : RandomNumber  Seed=seed  SampleTime=Ts
  Zero-Order Hold : ZeroOrderHold  SampleTime=Ts
  Out_1 : Outport
  wires:
  White Noise/1 -> Zero-Order Hold/1
  Gain/1 -> Out_1/1
  Zero-Order Hold/1 -> Gain/1

== system wt_blockset_v3/Mechanical Components/Wind Model SB-1/White Noise_2 ==
  Gain : Gain  Gain=[sqrt(Cov)]/[sqrt(Ts)]  SaturateOnIntegerOverflow=on
  White Noise : RandomNumber  Seed=seed  SampleTime=Ts
  Zero-Order Hold : ZeroOrderHold  SampleTime=Ts
  Out_1 : Outport
  wires:
  White Noise/1 -> Zero-Order Hold/1
  Gain/1 -> Out_1/1
  Zero-Order Hold/1 -> Gain/1

== system wt_blockset_v3/Mechanical Components/Wind Model SB-1/White Noise_3 ==
  Gain : Gain  Gain=[sqrt(Cov)]/[sqrt(Ts)]  SaturateOnIntegerOverflow=on
  White Noise : RandomNumber  Seed=seed  SampleTime=Ts
  Zero-Order Hold : ZeroOrderHold  SampleTime=Ts
  Out_1 : Outport
  wires:
  White Noise/1 -> Zero-Order Hold/1
  Gain/1 -> Out_1/1
  Zero-Order Hold/1 -> Gain/1

== system wt_blockset_v3/Mechanical Components/Wind Model SB-2/3rd_Harmonic_Filter1 ==
  avg_wind : Inport  Port=1  LatchInput=off
  in_1 : Inport  Port=2  LatchInput=off
  3rd harmonic Filter : Subsystem
  Unit Delay : UnitDelay  SampleTime=T_sample
  out_1 : Outport
  wires:
  Unit Delay/1 -> 3rd harmonic Filter/2(In)
  in_1/1 -> Unit Delay/1
  avg_wind/1 -> 3rd harmonic Filter/1(avg_wind)
  3rd harmonic Filter/1(Out) -> out_1/1

== system wt_blockset_v3/Mechanical Components/Wind Model SB-2/3rd_Harmonic_Filter2 ==
  avg_wind : Inport  Port=1  LatchInput=off
  in_1 : Inport  Port=2  LatchInput=off
  3rd harmonic Filter : Subsystem
  Unit Delay : UnitDelay  SampleTime=T_sample
  out_1 : Outport
  wires:
  3rd harmonic Filter/1(Out) -> out_1/1
  avg_wind/1 -> 3rd harmonic Filter/1(avg_wind)
  in_1/1 -> Unit Delay/1
  Unit Delay/1 -> 3rd harmonic Filter/2(In)

== system wt_blockset_v3/Mechanical Components/Wind Model SB-2/Kaimal_Filter_1 ==
  in_1 : Inport  Port=1  LatchInput=off
  avg_wind : Inport  Port=2  LatchInput=off
  Fcn : Fcn  Expr=turb_int*sqrt(L*u(1))/100/sqrt(2)
  Kaimal Filter : Subsystem
  Product : Product  SaturateOnIntegerOverflow=on
  Unit Delay : UnitDelay  SampleTime=T_sample
  out_1 : Outport
  wires:
  Unit Delay/1 -> Kaimal Filter/2(In)
  in_1/1 -> Unit Delay/1
  avg_wind/1 -> Kaimal Filter/1(avg_wind), Fcn/1
  Fcn/1 -> Product/1
  Kaimal Filter/1(Out) -> Product/2
  Product/1 -> out_1/1

== system wt_blockset_v3/Mechanical Components/Wind Model SB-2/Kaimal_Filter_2 ==
  avg_wind : Inport  Port=1  LatchInput=off
  in_1 : Inport  Port=2  LatchInput=off
  Fcn : Fcn  Expr=turb_int*sqrt(L*u(1))/100/sqrt(2)
  Kaimal Filter : Subsystem
  Product : Product  SaturateOnIntegerOverflow=on
  Unit Delay : UnitDelay  SampleTime=T_sample
  out_1 : Outport
  wires:
  Product/1 -> out_1/1
  Kaimal Filter/1(Out) -> Product/2
  Fcn/1 -> Product/1
  avg_wind/1 -> Fcn/1, Kaimal Filter/1(avg_wind)
  in_1/1 -> Unit Delay/1
  Unit Delay/1 -> Kaimal Filter/2(In)

== system wt_blockset_v3/Mechanical Components/Wind Model SB-2/Kaimal_Filter_3 ==
  avg_wind : Inport  Port=1  LatchInput=off
  in_1 : Inport  Port=2  LatchInput=off
  Fcn : Fcn  Expr=turb_int*sqrt(L*u(1))/100/sqrt(2)
  Kaimal Filter : Subsystem
  Product : Product  SaturateOnIntegerOverflow=on
  Unit Delay : UnitDelay  SampleTime=T_sample
  out_1 : Outport
  wires:
  Unit Delay/1 -> Kaimal Filter/2(In)
  in_1/1 -> Unit Delay/1
  avg_wind/1 -> Kaimal Filter/1(avg_wind), Fcn/1
  Fcn/1 -> Product/1
  Kaimal Filter/1(Out) -> Product/2
  Product/1 -> out_1/1

== system wt_blockset_v3/Mechanical Components/Wind Model SB-2/White Noise_1 ==
  Gain : Gain  Gain=[sqrt(Cov)]/[sqrt(Ts)]  SaturateOnIntegerOverflow=on
  White Noise : RandomNumber  Seed=seed  SampleTime=Ts
  Zero-Order Hold : ZeroOrderHold  SampleTime=Ts
  Out_1 : Outport
  wires:
  Zero-Order Hold/1 -> Gain/1
  Gain/1 -> Out_1/1
  White Noise/1 -> Zero-Order Hold/1

== system wt_blockset_v3/Mechanical Components/Wind Model SB-2/White Noise_2 ==
  Gain : Gain  Gain=[sqrt(Cov)]/[sqrt(Ts)]  SaturateOnIntegerOverflow=on
  White Noise : RandomNumber  Seed=seed  SampleTime=Ts
  Zero-Order Hold : ZeroOrderHold  SampleTime=Ts
  Out_1 : Outport
  wires:
  Zero-Order Hold/1 -> Gain/1
  Gain/1 -> Out_1/1
  White Noise/1 -> Zero-Order Hold/1

== system wt_blockset_v3/Mechanical Components/Wind Model SB-2/White Noise_3 ==
  Gain : Gain  Gain=[sqrt(Cov)]/[sqrt(Ts)]  SaturateOnIntegerOverflow=on
  White Noise : RandomNumber  Seed=seed  SampleTime=Ts
  Zero-Order Hold : ZeroOrderHold  SampleTime=Ts
  Out_1 : Outport
  wires:
  Zero-Order Hold/1 -> Gain/1
  Gain/1 -> Out_1/1
  White Noise/1 -> Zero-Order Hold/1

== system wt_blockset_v3/Mechanical Components/Wind Model SB-2/ZERO_Harmonic_Filter ==
  in_1 : Inport  Port=1  LatchInput=off
  avg_wind : Inport  Port=2  LatchInput=off
  Unit Delay : UnitDelay  SampleTime=T_sample
  ZERO harmonic Filter : Subsystem
  out_1 : Outport
  wires:
  ZERO harmonic Filter/1(Out) -> out_1/1
  avg_wind/1 -> ZERO harmonic Filter/1(avg_wind)
  in_1/1 -> Unit Delay/1
  Unit Delay/1 -> ZERO harmonic Filter/2(In)

== system wt_blockset_v3/Mechanical Components/Wind Model ZA-1/Band Limited White Noise ==
  Gain : Gain  Gain=sqrt(noise/T_sample)  SaturateOnIntegerOverflow=on
  S-Function : S-Function  FunctionName=rngen  Parameters=seed
  Zero-Order Hold : ZeroOrderHold  SampleTime=T_sample
  wn : Outport
  wires:
  S-Function/1 -> Zero-Order Hold/1
  Zero-Order Hold/1 -> Gain/1
  Gain/1 -> wn/1

== system wt_blockset_v3/Mechanical Components/Wind Model ZA-1/Band Limited White Noise1 ==
  Gain : Gain  Gain=sqrt(noise/T_sample)  SaturateOnIntegerOverflow=on
  S-Function : S-Function  FunctionName=rngen  Parameters=seed
  Zero-Order Hold : ZeroOrderHold  SampleTime=T_sample
  wn : Outport
  wires:
  Gain/1 -> wn/1
  Zero-Order Hold/1 -> Gain/1
  S-Function/1 -> Zero-Order Hold/1

== system wt_blockset_v3/Mechanical Components/Wind Model ZA-1/Band Limited White Noise2 ==
  Gain : Gain  Gain=sqrt(noise/T_sample)  SaturateOnIntegerOverflow=on
  S-Function : S-Function  FunctionName=rngen  Parameters=seed
  Zero-Order Hold : ZeroOrderHold  SampleTime=T_sample
  wn : Outport
  wires:
  S-Function/1 -> Zero-Order Hold/1
  Zero-Order Hold/1 -> Gain/1
  Gain/1 -> wn/1

== system wt_blockset_v3/Mechanical Components/Wind Model ZA-1/Kaimal_Filter_1 ==
  in_1 : Inport  Port=1  LatchInput=off
  Gain : Gain  Gain=trans/sqrt(2)  SaturateOnIntegerOverflow=on
  Transfer Fcn : TransferFcn  Numerator=[0.0182*c^2 1.3653*c 0.9846]  Denominator=[1.3463*c^2 3.7593*c 1]
  Unit Delay : UnitDelay  SampleTime=T_sample
  out_1 : Outport
  wires:
  Unit Delay/1 -> Transfer Fcn/1
  Gain/1 -> out_1/1
  in_1/1 -> Unit Delay/1
  Transfer Fcn/1 -> Gain/1
